simulink model "leadCar"  (R2024b)
settings: Solver=FixedStepAuto  StartTime=0.0  StopTime=80.0  RelTol=1e-3
settings Model: Creator=deyun  LastModifiedBy=deyun
settings OptimizationCC: DefaultParameterBehavior=Inlined  EnhancedBackFolding=on  PassReuseOutputArgsAs=Individual arguments  ZeroExternalMemoryAtStartup=off  ZeroInternalMemoryAtStartup=off  OptimizeBlockOrder=speed  DifferentSizesBufferReuse=on  OptimizationCustomize=off  EfficientTunableParamExpr=on
settings DebuggingCC: ParameterTunabilityLossMsg=error
settings HardwareCC: ProdBitPerLong=64  ProdHWDeviceType=Apple->ARM64
settings SFSimCC: MATLABDynamicMemAlloc=off
settings RTWCC: Description=Embedded Coder  SystemTargetFile=ert.tlc  GenCodeOnly=on  PackageGeneratedCodeAndArtifacts=on  TemplateMakefile=ert_default_tmf  TargetLang=C++
settings CodeAppCC: ForceParamTrailComments=on  IgnoreCustomStorageClasses=off  OperatorAnnotations=on  SimulinkDataObjDesc=on  SFDataObjDesc=on  InsertBlockDesc=on
settings ERTTargetCC: TargetLangStandard=C++14 (ISO)  GenerateSampleERTMain=on  CodeInterfacePackaging=C++ class  SupportContinuousTime=on  RootIOFormat=Structure reference  ERTCustomFileTemplate=example_file_process.tlc

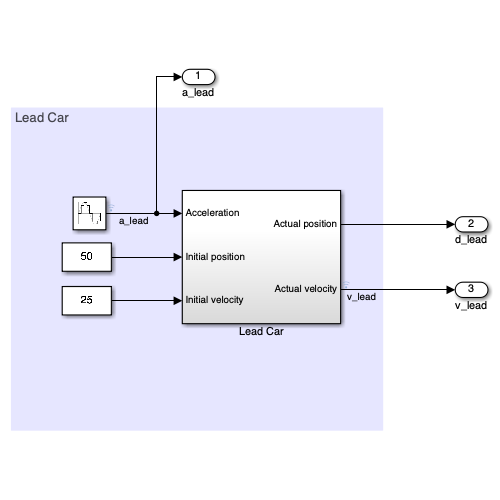
[thumbnail: Simulink's stored preview of the top-level diagram]
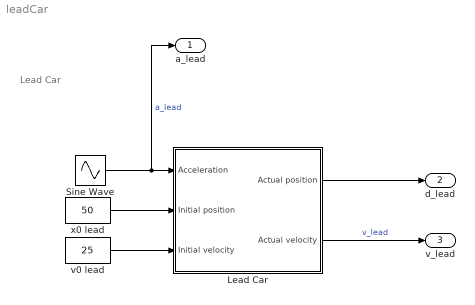
== system leadCar ==
  note: Lead Car
  Lead Car : Subsystem
  Sine Wave : Sin  Amplitude=0.6  Frequency=0.2  SampleTime=0.1
  v0 lead : Constant  Value=25  SampleTime=0.1
  x0 lead : Constant  Value=50  SampleTime=0.1
  a_lead : Outport
  d_lead : Outport  Port=2
  v_lead : Outport  Port=3
  wires:
  Lead Car/1(Actual position) -> d_lead/1
  Sine Wave/1 -> a_lead/1, Lead Car/1(Acceleration)  "a_lead"
  Lead Car/2(Actual velocity) -> v_lead/1  "v_lead"
  x0 lead/1 -> Lead Car/2(Initial position)
  v0 lead/1 -> Lead Car/3(Initial velocity)

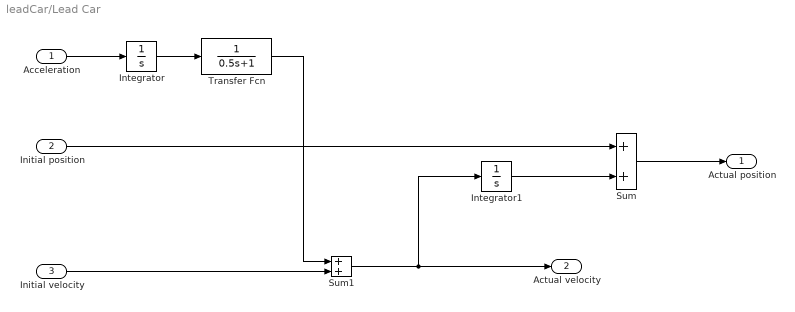
== system leadCar/Lead Car ==
  Acceleration : Inport
  Initial position : Inport  Port=2
  Initial velocity : Inport  Port=3
  Integrator : Integrator
  Integrator1 : Integrator
  Sum : Sum
  Sum1 : Sum
  Transfer Fcn : TransferFcn  Denominator=[0.5 1]
  Actual position : Outport  VectorParamsAs1DForOutWhenUnconnected=off
  Actual velocity : Outport  Port=2  VectorParamsAs1DForOutWhenUnconnected=off
  wires:
  Transfer Fcn/1 -> Sum1/1
  Initial velocity/1 -> Sum1/2
  Sum/1 -> Actual position/1
  Integrator/1 -> Transfer Fcn/1
  Sum1/1 -> Integrator1/1, Actual velocity/1
  Acceleration/1 -> Integrator/1
  Initial position/1 -> Sum/1
  Integrator1/1 -> Sum/2
